simulink model "tp3_practica1"  (R2025b)
settings: Solver=VariableStepAuto  StartTime=0.0  StopTime=200  RelTol=1e-3
undefined symbols (not defined in the file or in its folder): dspblkCoreblockFVToolHelper, gcbh

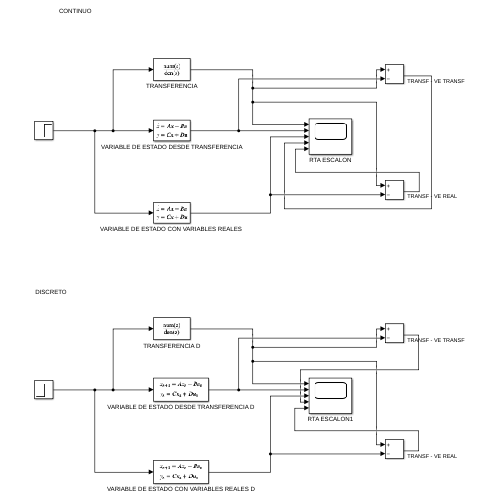
[thumbnail: Simulink's stored preview of the top-level diagram]
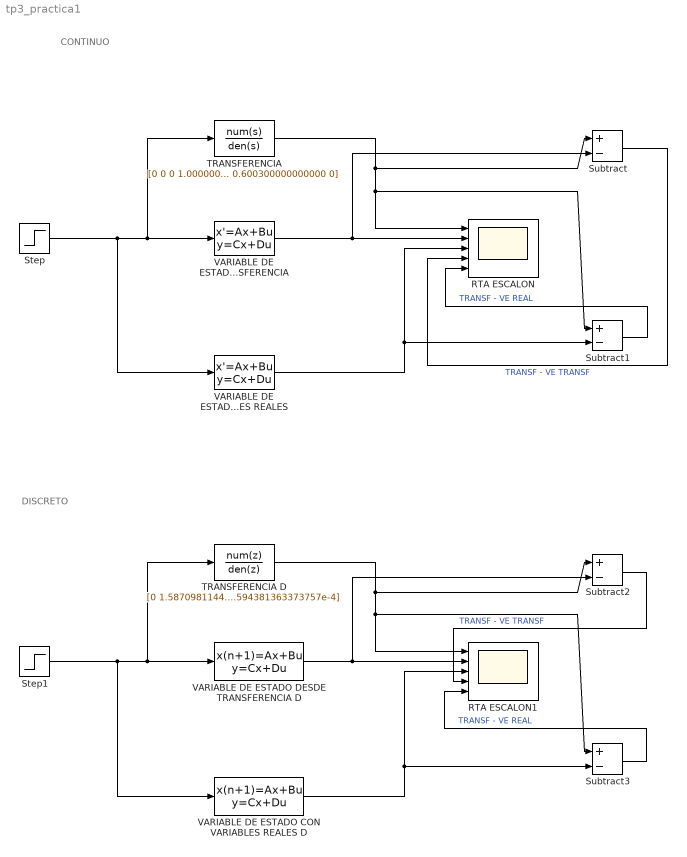
== system tp3_practica1 ==
  note: CONTINUO
  note: DISCRETO
  RTA ESCALON : Scope  NumInputPorts=5
      settings: ActiveDisplayYMinimum=-0.031391728519890139  ActiveDisplayYMaximum=0.2825255566790113  DataLoggingVariableName=ScopeData3
  RTA ESCALON1 : Scope  NumInputPorts=5
      settings: ActiveDisplayYMinimum=-0.031345935751424317  ActiveDisplayYMaximum=0.28211342176281889
  Step : Step  Time=0  SampleTime=0
  Step1 : Step  Time=0  SampleTime=0
  Subtract{,1..3} (4 alike) : Sum  Inputs=+-
  TRANSFERENCIA : TransferFcn  Numerator=[0 0 0 1.000000000000000e-03]  Denominator=[4.214000000000000 30.114041999999998 0.600300000000000 0]
  TRANSFERENCIA D : DiscreteTransferFcn  LoadFcn=dspblkCoreblockFVToolHelper(gcbh,'load');  Numerator=[0 1.587098114499472e-5 2.404465224969516e-5 6.336036425624988e-7]  Denominator=[1 -1.978426373061843 0.978785811198180 -3.594381363373757e-4]
      settings: CopyFcn=dspblkCoreblockFVToolHelper(gcbh,'copy');  DeleteFcn=dspblkCoreblockFVToolHelper(gcbh,'close');  ModelCloseFcn=dspblkCoreblockFVToolHelper(gcbh,'close');  PreSaveFcn=dspblkCoreblockFVToolHelper(gcbh,'presave');  PostSaveFcn=dspblkCoreblockFVToolHelper(gcbh,'postsave');  CloseFcn=dspblkCoreblockFVToolHelper(gcbh,'close');
  "VARIABLE DE ESTADO CON VARIABLES REALES " : StateSpace  A=[0 1 0;0 -0.003332225913621 0.166112956810631;0 -0.714285714285714 -7.142857142857143]  B=[0;0;1.428571428571429]  C=[0.001 0 0]  D=0  InitialCondition=0
  VARIABLE DE ESTADO CON VARIABLES REALES D : DiscreteStateSpace  A=[1 1.099843354794288 0.022376553702284;0 0.980353949318994 0.022852733446660;0 -0.098276384713722 -0.001924225638413]  B=[0.015870171846444;0.031967144619082;0.197193651977604]  C=[1e-03 0 0]  D=0  SampleTime=1.109817844007972
  VARIABLE DE ESTADO DESDE TRANSFERENCIA : StateSpace  A=[0 1 0;0 0 1;0 -0.142453725676317 -7.146189368770763]  B=[0;0;2.373042240151875e-04]  C=[1 0 0]  D=0  InitialCondition=0
  VARIABLE DE ESTADO DESDE TRANSFERENCIA D : DiscreteStateSpace  A=[0 1 0;0 0 1;0.000359438136337 -0.978785811198180 1.978426373061843]  B=[0;0;1]  C=[6.336036425624988e-7 2.404465224969516e-5 1.587098114499472e-5]  D=0  SampleTime=1.109817844007972
  wires:
  Step/1 -> TRANSFERENCIA/1, VARIABLE DE ESTADO DESDE TRANSFERENCIA/1, "VARIABLE DE ESTADO CON VARIABLES REALES "/1
  TRANSFERENCIA/1 -> RTA ESCALON/1, Subtract1/1, Subtract/1
  VARIABLE DE ESTADO DESDE TRANSFERENCIA/1 -> Subtract/2, RTA ESCALON/2
  "VARIABLE DE ESTADO CON VARIABLES REALES "/1 -> Subtract1/2, RTA ESCALON/3
  Subtract/1 -> RTA ESCALON/4  "TRANSF - VE TRANSF"
  Subtract1/1 -> RTA ESCALON/5  "TRANSF - VE REAL"
  VARIABLE DE ESTADO CON VARIABLES REALES D/1 -> Subtract3/2, RTA ESCALON1/3
  Subtract2/1 -> RTA ESCALON1/4  "TRANSF - VE TRANSF"
  Subtract3/1 -> RTA ESCALON1/5  "TRANSF - VE REAL"
  TRANSFERENCIA D/1 -> RTA ESCALON1/1, Subtract3/1, Subtract2/1
  VARIABLE DE ESTADO DESDE TRANSFERENCIA D/1 -> Subtract2/2, RTA ESCALON1/2
  Step1/1 -> VARIABLE DE ESTADO CON VARIABLES REALES D/1, VARIABLE DE ESTADO DESDE TRANSFERENCIA D/1, TRANSFERENCIA D/1
